simulink model "Adaptive_PTC_7dof"  (R2024a)
settings: Solver=ode4  StartTime=0.0  StopTime=7  FixedStep=0.01  RelTol=1e-3
model workspace (MAT data in the model file):
  e2 : Simulink.Signal (value not decoded)
undefined symbols (not defined in the file): D
libraries: aerolibconvert2 x16
(part 2 of 2)

== matlab function Adaptive_PTC_7dof/MATLAB Function ==
  data: Fx input; Fy input; Fz input; theta1 input; theta2 input; theta3 input; theta4 input; x_dot input; y_dot input; l1_dot input; theta1_dot input; theta2_dot input; theta3_dot input; theta4_dot input; m1 input; m2 input; M1 input; M2 input; l1 input; l2 input; q_ddot output size=[7 1]; Frx input; Fry input; Frz input
function q_ddot   = fcn(Fx, Fy, Fz, theta1, theta2, theta3, theta4,...
    x_dot, y_dot, l1_dot, theta1_dot, theta2_dot, theta3_dot, theta4_dot,...
    m1, m2, M1, M2, l1, l2, Frx, Fry, Frz)

g = 9.8;


% Mass matrix M(q)
M = zeros(7, 7);

% Define M matrix elements
M(1,1) = M1 + m1 + m2;
M(1,2) = 0;
M(1,3) = (m1 + m2) * sin(theta1) * cos(theta2);
M(1,4) = (m1 + m2) * l1 * cos(theta1) * cos(theta2);
M(1,5) = -(m1 + m2) * l1 * sin(theta1) * sin(theta2);
M(1,6) = m2 * l2 * cos(theta3) * cos(theta4);
M(1,7) = -m2 * l2 * sin(theta3) * sin(theta4);

M(2,1) = 0;
M(2,2) = M2 + m1 + m2;
M(2,3) = (m1 + m2) * sin(theta2);
M(2,4) = 0;
M(2,5) = (m1 + m2) * l1 * cos(theta2);
M(2,6) = 0;
M(2,7) = m2 * l2 * cos(theta4);

M(3,1) = (m1 + m2) * sin(theta1) * cos(theta2);
M(3,2) = (m1 + m2) * sin(theta2);
M(3,3) = m1 + m2;
M(3,4) = 0;
M(3,5) = 0;
M(3,6) = m2 * l2 * cos(theta2) * cos(theta4) * sin(theta1 - theta3);
M(3,7) = m2 * l2 * (sin(theta2) * cos(theta4) - cos(theta2) * sin(theta4) * cos(theta1 - theta3));

M(4,1) = (m1 + m2) * l1 * cos(theta1) * cos(theta2);
M(4,2) = 0;
M(4,3) = 0;
M(4,4) = (m1 + m2) * l1^2 * cos(theta2)^2;
M(4,5) = 0;
M(4,6) = m2*l1*l2*cos(theta2)*cos(theta4)*cos(theta1-theta3);
M(4,7) = m2*l1*l2*cos(theta2)*sin(theta4)*sin(theta1 - theta3);

M(5,1) = -(m1 + m2) * l1 * sin(theta1) * sin(theta2);
M(5,2) = (m1 + m2) * l1 * cos(theta2);
M(5,3) = 0;
M(5,4) = 0;
M(5,5) = (m1 + m2) * l1^2;
M(5,6) = -m2 * l1 * l2 * sin(theta2) * cos(theta4) * sin(theta1 - theta3);
M(5,7) = m2 * l1 * l2 * (cos(theta2) * cos(theta4) + sin(theta2) * sin(theta4) * cos(theta1 - theta3));

M(6,1) = m2 * l2 * cos(theta3) * cos(theta4);
M(6,2) = 0;
M(6,3) = m2 * l2 * cos(theta2) * cos(theta4) * sin(theta1 - theta3);
M(6,4) = m2*l1*l2*cos(theta2)*cos(theta4)*cos(theta1-theta3);
M(6,5) = -m2 * l1 * l2 * sin(theta2) * cos(theta4) * sin(theta1 - theta3);
M(6,6) = m2 * l2^2 * cos(theta4)^2;
M(6,7) = 0;

M(7,1) = -m2 * l2 * sin(theta3) * sin(theta4);
M(7,2) = m2 * l2 * cos(theta4);
M(7,3) = m2 * l2 * (sin(theta2) * cos(theta4) - cos(theta2) * sin(theta4) * cos(theta1 - theta3));
M(7,4) = m2*l1*l2*cos(theta2)*sin(theta4)*sin(theta1 - theta3);
M(7,5) = m2 * l1 * l2 * (cos(theta2) * cos(theta4) + sin(theta2) * sin(theta4) * cos(theta1 - theta3));
M(7,6) = 0;
M(7,7) = m2 * l2^2;

% Coriolis matrix C(q, dq)
C = zeros(7, 7);

% Define C matrix elements
C(1,3) = (m1 + m2) * (cos(theta1) * cos(theta2) * theta1_dot - sin(theta1) * sin(theta2) * theta2_dot);
C(1,4) = (m1 + m2) * (cos(theta1) * cos(theta2) * l1_dot - l1 * sin(theta1) * sin(theta2) * theta1_dot - l1 * cos(theta1) * sin(theta2) * theta2_dot);
C(1,5) = -(m1 + m2) * (sin(theta1) * sin(theta2) * l1_dot + l1 * cos(theta1) * sin(theta2) * theta1_dot + l1 * sin(theta1) * cos(theta2) * theta2_dot);
C(1,6) = -m2 * l2 * (sin(theta3) * cos(theta4) * theta3_dot + cos(theta3) * sin(theta4) * theta4_dot);
C(1,7) = -m2 * l2 * (cos(theta3) * sin(theta4) * theta3_dot + sin(theta3) * cos(theta4) * theta4_dot);

C(2,3) = (m1 + m2) * cos(theta2) * theta2_dot;
C(2,5) = (m1 + m2) * (cos(theta2) * l1_dot - l1 * sin(theta2) * theta2_dot);
C(2,7) = -m2 * l2 * sin(theta4) * theta4_dot;

C(3,4) = -(m1 + m2) * l1 * cos(theta2)^2 * theta1_dot;
C(3,5) = -(m1 + m2) * l1 * theta2_dot;
C(3,6) = -m2 * l2 * (cos(theta2) * cos(theta4) * cos(theta1 - theta3) * theta3_dot + cos(theta2) * sin(theta4) * sin(theta1 - theta3) * theta4_dot);
C(3,7) = -m2 * l2 * (cos(theta2) * sin(theta4) * theta3_dot + sin(theta2) * sin(theta4) * theta4_dot + cos(theta2) * cos(theta4) * cos(theta1 - theta3) * theta4_dot);

C(4,3) = (m1 + m2) * l1 * cos(theta2)^2 * theta1_dot;
C(4,4) = (m1 + m2) * (l1 * cos(theta2)^2 * l1_dot - l1^2 * sin(theta2) * cos(theta2) * theta2_dot);
C(4,5) = -(m1 + m2) * l1^2 * sin(theta2) * cos(theta2) * theta1_dot;
C(4,6) = m2 * l1 * l2 * (cos(theta2) * cos(theta4) * sin(theta1 - theta3) * theta3_dot + cos(theta2) * sin(theta4) * cos(theta1 - theta3) * theta4_dot);
C(4,7) = m2 * l1 * l2 * (cos(theta2) * cos(theta4) * sin(theta1 - theta3) * theta4_dot + cos(theta2) * sin(theta4) * cos(theta1 - theta3) * theta3_dot);

C(5,3) = (m1 + m2) * l1 * theta2_dot;
C(5,4) = (m1 + m2) * l1^2 * sin(theta2) * cos(theta2) * theta1_dot;
C(5,5) = (m1 + m2) * l1 * l1_dot;
C(5,6) = m2 * l1 * l2 * (sin(theta2) * cos(theta4) * cos(theta1 - theta3) * theta3_dot + sin(theta2) * sin(theta4) * sin(theta1 - theta3) * theta4_dot);
C(5,7) = m2 * l1 * l2 * (sin(theta2) * sin(theta4) * sin(theta1 - theta3) * theta3_dot + sin(theta2) * cos(theta4) * cos(theta1 - theta3) * theta4_dot ...
    - cos(theta2) * sin(theta4) * theta4_dot);

C(6,3) = m2 * l2 * (cos(theta2) * cos(theta4) * cos(theta1 - theta3) * theta1_dot - sin(theta2) * cos(theta4) * sin(theta1 - theta3) * theta2_dot);
C(6,4) = m2 * l2 * (cos(theta2) * cos(theta4) * cos(theta1 - theta3) * l1_dot - l1 * cos(theta2) * cos(theta4) * sin(theta1 - theta3) ...
    * theta1_dot - l1 * sin(theta2) * cos(theta4) * cos(theta1 - theta3) * theta2_dot);
C(6,5) = -m2 * l2 * (sin(theta2) * cos(theta4) * sin(theta1 - theta3) * l1_dot + l1 * sin(theta2) * cos(theta4) * cos(theta1 - theta3) ...
    * theta1_dot + l1 * cos(theta2) * cos(theta4) * sin(theta1 - theta3) * theta2_dot);
C(6,6) = -m2 * l2^2 * sin(theta4) * cos(theta4) * theta4_dot;
C(6,7) = -m2 * l2^2 * sin(theta4) * cos(theta4) * theta3_dot;

C(7,3) = m2 * l2 * (cos(theta2) * sin(theta4) * sin(theta1 - theta3) * theta1_dot + sin(theta2) * sin(theta4) * cos(theta1 - theta3) * theta2_dot ...
    + cos(theta2) * cos(theta4) * theta2_dot);
C(7,4) = m2 * l2 * (cos(theta2) * sin(theta4) * sin(theta1 - theta3) * l1_dot + l1 * cos(theta2) * sin(theta4) * cos(theta1 - theta3) ...
    * theta1_dot - l1 * sin(theta2) * sin(theta4) * sin(theta1 - theta3)*theta2_dot);
C(7,5) = m2 * l2 * (cos(theta2)*cos(theta4)*l1_dot + sin(theta2)*sin(theta4)*cos(theta1 - theta3)*l1_dot - l1 * sin(theta2)*sin(theta4)...
    *sin(theta1 - theta3)*theta1_dot + l1*cos(theta2)*sin(theta4)*cos(theta1 - theta3)*theta2_dot - l1*sin(theta2)*cos(theta4)*theta2_dot);
C(7,6) = m2 * l2^2 * sin(theta4) * cos(theta4) * theta3_dot;

% Gravity with friction matrix
G = zeros(7, 1);

% Define G matrix elements
G(1,1) = 0;
G(2,1) = 0;
G(3,1) = - (m1 + m2) * g * cos(theta1) * cos(theta2);
% G(3,1) = 0;
G(4,1) = (m1 + m2) * g * l1 * sin(theta1) * cos(theta2);
G(5,1) = (m1 + m2) * g * l1 * cos(theta1) * sin(theta2);
G(6,1) = m2 * g * l2 * sin(theta3) * cos(theta4);
G(7,1) = m2 * g * l2 * cos(theta3) * sin(theta4);


q_dot = [x_dot; y_dot; l1_dot; theta1_dot; theta2_dot; theta3_dot; theta4_dot];
tau = [Fx; Fy; Fz; 0; 0; 0; 0];
D = tau - C*q_dot - G;

q_ddot = M\D;

end
